simulink model "CSTR_MalhaFechada"  (R2021a)
settings: Solver=VariableStepAuto  StartTime=0.0  StopTime=tsim  RelTol=1e-3
values from neighbouring files (symbols this model uses):
  caf = 10    [mainCSTR.m]    (also in mainCSTR_control.m; mainControlCSTR.m; simulation_04_04_2024.mat)
  deltaE = 11843    [mainCSTR.m]    (also in mainCSTR_control.m; mainControlCSTR.m; simulation_04_04_2024.mat)
  deltaH = 5960    [mainCSTR.m]    (also in mainCSTR_control.m; mainControlCSTR.m; simulation_04_04_2024.mat)
  k0 = 9703*3600    (= 34930800)    [mainCSTR.m]    (also in mainCSTR_control.m; mainControlCSTR.m; simulation_04_04_2024.mat)
  R = 1.987    [mainCSTR.m]    (also in mainCSTR_control.m; mainControlCSTR.m; rga.m = pinv(G.').*G; simulation_04_04_2024.mat)
  rhocp = 500    [mainCSTR.m]    (also in mainCSTR_control.m; mainControlCSTR.m; simulation_04_04_2024.mat)
  Tf = 298    [mainCSTR.m]    (also in mainCSTR_control.m; mainControlCSTR.m; simulation_04_04_2024.mat)
  Ts = 0.1    [mainCSTR_control.m]    (also in mainControlCSTR.m; wandb.m = 0.5)
  UAoV = 150    [mainCSTR.m]    (also in mainCSTR_control.m; mainControlCSTR.m; simulation_04_04_2024.mat)
  x0model = [5, 350]    [mainCSTR.m]    (also in mainCSTR_control.m = [8.5636  311.1710]; mainControlCSTR.m = [8.5636  311.1706]; simulation_04_04_2024.mat = [5 350])
libraries: pid_lib x2
settings Model: Creator=Aula  LastModifiedBy=Aula
settings DataIOCC: ReturnWorkspaceOutputs=off

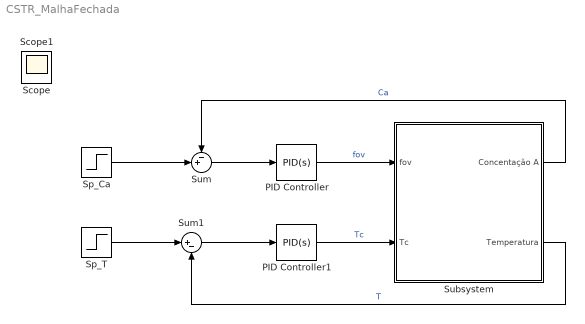
== system CSTR_MalhaFechada ==
  PID Controller : pid_lib/PID Controller  Controller=PID  Form=Parallel  TimeDomain=Continuous-time  UseExternalTs=off  SampleTime=-1  IntegratorMethod=Forward Euler  FilterMethod=Forward Euler  ControllerParametersSource=internal  P=1.20  I=1.22  D=0  UseFilter=on  N=100  TunerSelectOption=Transfer Function Based (PID Tuner App)  InitialConditionSource=internal  InitialConditionForIntegrator=1  InitialConditionForFilter=0  DifferentiatorICPrevScaledInput=0  ExternalReset=none  TrackingMode=off  Kt=1  LimitOutput=off  SatLimitsSource=internal  UpperSaturationLimit=inf  LowerSaturationLimit=-inf  LinearizeAsGain=on  AntiWindupMode=none  Kb=1  POutMin=[]  POutMax=[]  IOutMin=[]  IOutMax=[]  DOutMin=[]  DOutMax=[]  NOutMin=[]  NOutMax=[]  SumOutMin=[]  SumOutMax=[]  SaturationOutMin=[]  SaturationOutMax=[]  PParamMin=[]  PParamMax=[]  IParamMin=[]  IParamMax=[]  DParamMin=[]  DParamMax=[]  NParamMin=[]  NParamMax=[]  KbParamMin=[]  KbParamMax=[]  KtParamMin=[]  KtParamMax=[]  KbOutMin=[]  KbOutMax=[]  KtOutMin=[]  KtOutMax=[]  IntegratorOutMin=[]  IntegratorOutMax=[]  FilterOutMin=[]  FilterOutMax=[]  SumI1OutMin=[]  SumI1OutMax=[]  SumI2OutMin=[]  SumI2OutMax=[]  SumI3OutMin=[]  SumI3OutMax=[]  SumI4OutMin=[]  SumI4OutMax=[]  SumDOutMin=[]  SumDOutMax=[]  DifferentiatorOutMin=[]  DifferentiatorOutMax=[]  FilterDiffOutCoefMin=[]  FilterDiffOutCoefMax=[]  ReciprocalOutMin=[]  ReciprocalOutMax=[]  SumDenOutMin=[]  SumDenOutMax=[]  SumNumOutMin=[]  SumNumOutMax=[]  DivideOutMin=[]  DivideOutMax=[]  UdiffTsProdOutMin=[]  UdiffTsProdOutMax=[]  NTsProdOutMin=[]  NTsProdOutMax=[]  UintegralTsProdOutMin=[]  UintegralTsProdOutMax=[]  UngainTsProdOutMin=[]  UngainTsProdOutMax=[]  IntegratorContinuousStateAttributes=''  IntegratorStateMustResolveToSignalObject=off  IntegratorRTWStateStorageClass=Auto  FilterContinuousStateAttributes=''  FilterStateMustResolveToSignalObject=off  FilterRTWStateStorageClass=Auto  ParallelPVariant=InternalParameters  IdealPVariant=Disabled  IVariant=InternalParameters  DVariant=InternalParameters  IntegratorVariant=Continuous  SatVariant=Disabled  AWVariant=Passthrough  PCopyVariant=Disabled  TRVariant=Disabled  FdbkBlocksVariant=Forward  IdealPFdbkVariant=Disabled  SatFdbkVariant=Disabled  DerivativeFilterVariant=ContFilter  NVariant=InternalParameters  NCopyVariant=Disabled  FilterICVariant=InternalICsFilter  IntegratorICVariant=InternalICs  ExternalResetVariant=Disabled  TRSumVariant=Passthrough  SumFdbkVariant=Disabled  SumVariant=Sum_PID  TsampFilterVariant=InternalTs  TsampNgainVariant=Passthrough  TsampIntegralVariant=Passthrough  ExternalSaturationOutDataTypeStr=Inherit: Same as second input
  PID Controller1 : pid_lib/PID Controller  Controller=PID  Form=Parallel  TimeDomain=Continuous-time  UseExternalTs=off  SampleTime=-1  IntegratorMethod=Forward Euler  FilterMethod=Forward Euler  ControllerParametersSource=internal  P=9.8  I=8.5  D=0  UseFilter=on  N=100  TunerSelectOption=Transfer Function Based (PID Tuner App)  InitialConditionSource=internal  InitialConditionForIntegrator=298  InitialConditionForFilter=0  DifferentiatorICPrevScaledInput=0  ExternalReset=none  TrackingMode=off  Kt=1  LimitOutput=off  SatLimitsSource=internal  UpperSaturationLimit=inf  LowerSaturationLimit=-inf  LinearizeAsGain=on  AntiWindupMode=none  Kb=1  POutMin=[]  POutMax=[]  IOutMin=[]  IOutMax=[]  DOutMin=[]  DOutMax=[]  NOutMin=[]  NOutMax=[]  SumOutMin=[]  SumOutMax=[]  SaturationOutMin=[]  SaturationOutMax=[]  PParamMin=[]  PParamMax=[]  IParamMin=[]  IParamMax=[]  DParamMin=[]  DParamMax=[]  NParamMin=[]  NParamMax=[]  KbParamMin=[]  KbParamMax=[]  KtParamMin=[]  KtParamMax=[]  KbOutMin=[]  KbOutMax=[]  KtOutMin=[]  KtOutMax=[]  IntegratorOutMin=[]  IntegratorOutMax=[]  FilterOutMin=[]  FilterOutMax=[]  SumI1OutMin=[]  SumI1OutMax=[]  SumI2OutMin=[]  SumI2OutMax=[]  SumI3OutMin=[]  SumI3OutMax=[]  SumI4OutMin=[]  SumI4OutMax=[]  SumDOutMin=[]  SumDOutMax=[]  DifferentiatorOutMin=[]  DifferentiatorOutMax=[]  FilterDiffOutCoefMin=[]  FilterDiffOutCoefMax=[]  ReciprocalOutMin=[]  ReciprocalOutMax=[]  SumDenOutMin=[]  SumDenOutMax=[]  SumNumOutMin=[]  SumNumOutMax=[]  DivideOutMin=[]  DivideOutMax=[]  UdiffTsProdOutMin=[]  UdiffTsProdOutMax=[]  NTsProdOutMin=[]  NTsProdOutMax=[]  UintegralTsProdOutMin=[]  UintegralTsProdOutMax=[]  UngainTsProdOutMin=[]  UngainTsProdOutMax=[]  IntegratorContinuousStateAttributes=''  IntegratorStateMustResolveToSignalObject=off  IntegratorRTWStateStorageClass=Auto  FilterContinuousStateAttributes=''  FilterStateMustResolveToSignalObject=off  FilterRTWStateStorageClass=Auto  ParallelPVariant=InternalParameters  IdealPVariant=Disabled  IVariant=InternalParameters  DVariant=InternalParameters  IntegratorVariant=Continuous  SatVariant=Disabled  AWVariant=Passthrough  PCopyVariant=Disabled  TRVariant=Disabled  FdbkBlocksVariant=Forward  IdealPFdbkVariant=Disabled  SatFdbkVariant=Disabled  DerivativeFilterVariant=ContFilter  NVariant=InternalParameters  NCopyVariant=Disabled  FilterICVariant=InternalICsFilter  IntegratorICVariant=InternalICs  ExternalResetVariant=Disabled  TRSumVariant=Passthrough  SumFdbkVariant=Disabled  SumVariant=Sum_PID  TsampFilterVariant=InternalTs  TsampNgainVariant=Passthrough  TsampIntegralVariant=Passthrough  ExternalSaturationOutDataTypeStr=Inherit: Same as second input
  Sp_Ca : Step  Time=2  Before=8.5636  After=8  SampleTime=0
  Sp_T : Step  Time=10  Before=311.1706  After=320  SampleTime=0
  Subsystem : Subsystem
      mask Display: image('cstr.png'); % Use "Edit Image" on toolstrip to change.
  Sum : Sum  Inputs=-+|
  Sum1 : Sum  Inputs=|+-
  Scope : Scope
  Scope1 : Scope
  wires:
  Subsystem/1(Concentação A) -> Sum/1  "Ca"
  Subsystem/2(Temperatura) -> Sum1/2  "T"
  PID Controller/1 -> Subsystem/1(fov)  "fov"
  PID Controller1/1 -> Subsystem/2(Tc)  "Tc"
  Sum/1 -> PID Controller/1
  Sum1/1 -> PID Controller1/1
  Sp_T/1 -> Sum1/1
  Sp_Ca/1 -> Sum/2

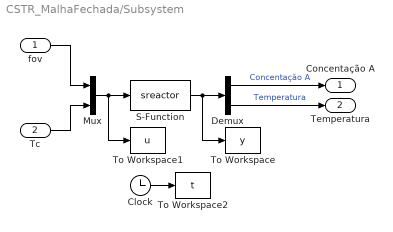
== system CSTR_MalhaFechada/Subsystem ==
  fov : Inport
  Tc : Inport  Port=2
  Clock : Clock
  Demux : Demux  Outputs=2
  Mux : Mux  Inputs=2
  S-Function : S-Function  FunctionName=sreactor  Parameters=x0model,k0,deltaE,R,caf,Tf,deltaH,rhocp,UAoV  SFunctionDeploymentMode=off  EnableBusSupport=off
  To Workspace : ToWorkspace  VariableName=y  SampleTime=Ts
  "To Workspace1 " : ToWorkspace  VariableName=u  SampleTime=Ts
  "To Workspace2 " : ToWorkspace  VariableName=t  SampleTime=Ts
  Concentação A : Outport
  Temperatura : Outport  Port=2
  wires:
  S-Function/1 -> To Workspace/1, Demux/1
  Clock/1 -> "To Workspace2 "/1
  fov/1 -> Mux/1
  Mux/1 -> "To Workspace1 "/1, S-Function/1
  Tc/1 -> Mux/2
  Demux/2 -> Temperatura/1  "Temperatura"
  Demux/1 -> Concentação A/1  "Concentação A"
